simulink model "MORUS_NELINEARNI_GA_NONTILTING"  (R2019a)
settings: Solver=FixedStepAuto  StartTime=0.0  StopTime=sim_time  RelTol=1e-3  EnableMultiTasking=on
values from neighbouring files (symbols this model uses):
  A_dis_calc = expm(kSamplingTime*A_continous_time)    [MPC_designer_X.m]    (also in NonTilting.m; RUN_simulation.m; Simulacija_MPC_YAW_NELINEARNI.m; Simulacija_MPC_Z.m)
  B_dis_calc = integral_exp_A * B_continous_time    [MPC_designer_X.m]    (also in NonTilting.m; RUN_simulation.m; Simulacija_MPC_YAW_NELINEARNI.m; Simulacija_MPC_Z.m)
  b_f = 4.56e-4    (= 0.000456)    [LinearizacijaMatrica.m]    (also in Linearizirane_matrice.mat; MPC_designer_X.m; NonTilting.m; RUN_simulation.m)
  b_m = 0.01    [LinearizacijaMatrica.m]    (also in Linearizirane_matrice.mat; MPC_designer_X.m; NonTilting.m; RUN_simulation.m)
  BETA = 0.0    (= 0)    [LinearizacijaMatrica.m]    (also in Linearizirane_matrice.mat; MPC_designer_X.m; NonTilting.m = 0.200712863979; RUN_simulation.m)
  g = 9.80665    [LinearizacijaMatrica.m]    (also in Linearizirane_matrice.mat; MPC_designer_X.m = 9.81; NonTilting.m = 9.81; RUN_simulation.m = 9.81)
  hover = 427.6233    [MPC_designer_X.m]    (also in NonTilting.m; RUN_simulation.m; Simulacija_MPC_YAW_NELINEARNI.m; Simulacija_MPC_Z.m)
  I_b_xx = 5.5268    [MPC_designer_X.m]    (also in NonTilting.m; RUN_simulation.m; Simulacija_MPC_YAW_NELINEARNI.m; Simulacija_MPC_Z.m)
  I_b_yy = 5.5268    [MPC_designer_X.m]    (also in NonTilting.m; RUN_simulation.m; Simulacija_MPC_YAW_NELINEARNI.m; Simulacija_MPC_Z.m)
  I_b_zz = 6.8854    [MPC_designer_X.m]    (also in NonTilting.m; RUN_simulation.m; Simulacija_MPC_YAW_NELINEARNI.m; Simulacija_MPC_Z.m)
  kSamplingTime = 0.810    (= 0.81)    [MPCDesigner_YAW.m]    (also in MPC_designer_X.m = 0.1; MPC_designer_Z.m; NonTilting.m = 0.015; RUN_simulation.m = 0.015)
  L = 0.84    [LinearizacijaMatrica.m]    (also in Linearizirane_matrice.mat; MPC_designer_X.m; NonTilting.m; RUN_simulation.m)
  m = 1.0    (= 1)    [LinearizacijaMatrica.m]    (also in Linearizirane_matrice.mat; MPC_designer_X.m; NonTilting.m; RUN_simulation.m)
  M = 34.8    [LinearizacijaMatrica.m]    (also in Linearizirane_matrice.mat; MPC_designer_X.m = 34; NonTilting.m = 34; RUN_simulation.m = 34)
  m_b = 30.8    [LinearizacijaMatrica.m]    (also in Linearizirane_matrice.mat; MPC_designer_X.m; NonTilting.m; RUN_simulation.m)
  odabir = 1    [MPC_designer_X.m]    (also in NonTilting.m; RUN_simulation.m; Simulacija_MPC_YAW_NELINEARNI.m; Simulacija_MPC_Z.m)
  Q = inv(diag([0.5800 4*kSamplingTime 0.5800 4*kSamplingTime 300 300 0.2 (0.2/3) 100 4])) * diag([0, 0, 0, 0, 0, 0, 1e5,0, 1e7, 0]) *inv(diag([0.5800 4*kSamplingTime 0.5800 4*kSamplingTime 300 300 0.2 (0.2/3.0) 100 4]))    [NonTilting.m]    (also in RUN_simulation.m = diag([ 0.135340000000000,0.002706800000000,  0.1353400, 0.00; Simulacija_MPC_YAW_NELINEARNI.m = diag([pop(5),pop(6),pop(5),pop(6), pop(7),pop(7),pop(8),pop(; Simulacija_MPC_Z.m = diag([pop(5),pop(6),pop(5),pop(6), pop(7),pop(7),pop(8),pop(; Simulacija_Roll.m = diag([pop(5),pop(6),pop(5),pop(6), pop(7),pop(7),pop(8),pop()
  R = inv(diag([0.5800 0.5800 300 300]))*diag([0, 0, 0, 0])*inv(diag([0.5800 0.5800 300 300]))    [NonTilting.m]    (also in RUN_simulation.m = diag([0.67670, 0.67670, 0.13534000, 0.13534000]); Simulacija_MPC_YAW_NELINEARNI.m = diag([pop(1),pop(1),pop(2),pop(2)]); Simulacija_MPC_Z.m = diag([pop(1),pop(1),pop(2),pop(2)]); Simulacija_Roll.m = diag([pop(1),pop(1),pop(2),pop(2)]))
  R_delta = inv(diag([0.5800 0.5800 300 300]))* diag([0,0,0,0])*inv(diag([0.5800 0.5800 300 300]))    [NonTilting.m]    (also in RUN_simulation.m = diag([0.738879858135067, 0.738879858135067, 0.00738879858135; Simulacija_MPC_YAW_NELINEARNI.m = diag([pop(3),pop(3),pop(4),pop(4)]); Simulacija_MPC_Z.m = diag([pop(3),pop(3),pop(4),pop(4)]); Simulacija_Roll.m = diag([pop(3),pop(3),pop(4),pop(4)]))
  T_r = 0.2    [LinearizacijaMatrica.m]    (also in Linearizirane_matrice.mat; MPC_designer_X.m; NonTilting.m; RUN_simulation.m)
  w_mm = 19.7845    [LinearizacijaMatrica.m]    (also in Linearizirane_matrice.mat; MPC_designer_X.m = 17; NonTilting.m = 17; RUN_simulation.m = 17)
  z_m = 0.05    [LinearizacijaMatrica.m]    (also in Linearizirane_matrice.mat; MPC_designer_X.m; NonTilting.m; RUN_simulation.m)
  z_r = 0.2    [LinearizacijaMatrica.m]    (also in Linearizirane_matrice.mat; MPC_designer_X.m; NonTilting.m; RUN_simulation.m)
  zeta_mm = 0.6544    [LinearizacijaMatrica.m]    (also in Linearizirane_matrice.mat; MPC_designer_X.m = 0.85; NonTilting.m = 0.85; RUN_simulation.m = 0.85)
libraries: simulink x8
(part 3 of 4)

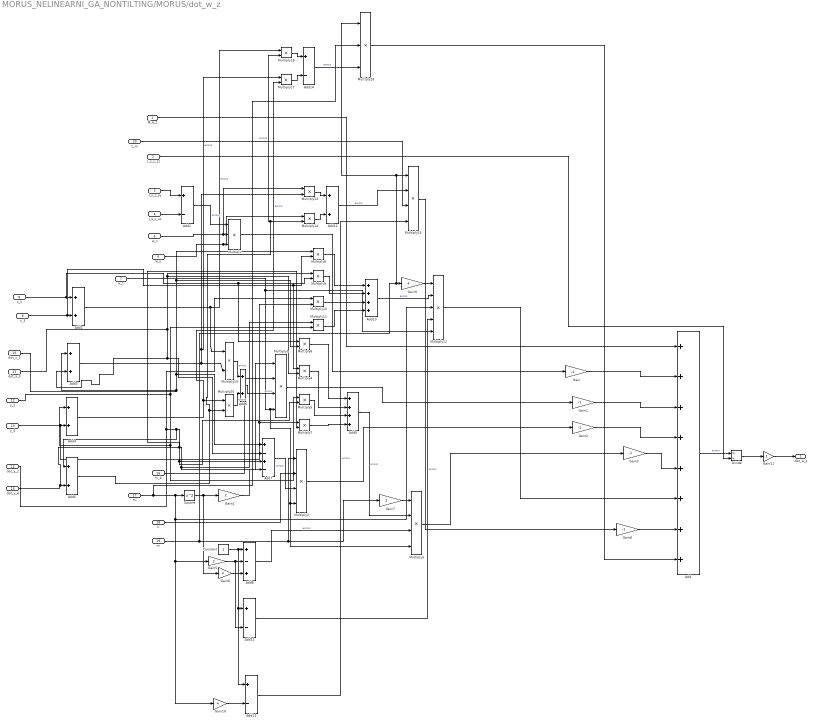
== system MORUS_NELINEARNI_GA_NONTILTING/MORUS/dot_w_z ==
  M_e_z : Inport
  I_s_c_zz : Inport  Port=2
  I_s_c_yy : Inport  Port=3
  I_s_c_xx : Inport  Port=4
  w_x : Inport  Port=5
  w_y : Inport  Port=6
  w_z : Inport  Port=7
  x_1 : Inport  Port=8
  x_3 : Inport  Port=9
  dot_x_1 : Inport  Port=10
  dot_x_3 : Inport  Port=11
  y_2 : Inport  Port=12
  y_4 : Inport  Port=13
  dot_y_2 : Inport  Port=14
  dot_y_4 : Inport  Port=15
  m_b : Inport  Port=16
  mi : Inport  Port=17
  L : Inport  Port=18
  m : Inport  Port=19
  z_m : Inport  Port=20
  Add : Sum  Inputs=++++++++  AccumDataTypeStr=double  OutDataTypeStr=double
  Add{1,11,13..14} (4 alike) : Sum  Inputs=+-  AccumDataTypeStr=double  OutDataTypeStr=double
  Add10 : Sum  Inputs=++++  AccumDataTypeStr=double  OutDataTypeStr=double
  Add{2..6,12} (6 alike) : Sum  AccumDataTypeStr=double  OutDataTypeStr=double
  Add7 : Sum  Inputs=+-+-  AccumDataTypeStr=double  OutDataTypeStr=double
  Add8 : Sum  Inputs=+-+  AccumDataTypeStr=double  OutDataTypeStr=double
  Add9 : Sum  Inputs=++++  AccumDataTypeStr=double  OutDataTypeStr=double
  Constant : Constant  OutDataTypeStr=double  SampleTime=-1
  Divide : Product  Inputs=*/  OutDataTypeStr=double
  Gain{,1..3,8} (5 alike) : Gain  Gain=-1
  Gain10 : Gain  Gain=4
  Gain11 : Gain
  Gain4 : Gain  Gain=2
  Gain5 : Gain  Gain=2
  Gain6 : Gain  Gain=4
  Gain7 : Gain  Gain=2
  Gain9 : Gain  Gain=4
  Multiply : Product  Inputs=3
  Multiply{1..3,15} (4 alike) : Product  Inputs=4
  Multiply{4..11,13..14,16..17,19..20} (14 alike) : Product
  Multiply12 : Product  Inputs=5
  Multiply18 : Product  Inputs=3
  Square : Math  Operator=square  SaturateOnIntegerOverflow=on
  dot_w_z : Outport  OutDataTypeStr=double
  wires:
  Add/1 -> Divide/1  "errors"
  I_s_c_zz/1 -> Divide/2
  Divide/1 -> Gain11/1
  M_e_z/1 -> Add/1
  I_s_c_xx/1 -> Add1/2
  I_s_c_yy/1 -> Add1/1
  Add1/1 -> Multiply/1  "errors"
  w_x/1 -> Multiply13/1, Multiply/2
  w_y/1 -> Multiply14/1, Multiply/3
  Gain/1 -> Add/2
  Gain2/1 -> Add/4
  Gain1/1 -> Add/3
  Gain3/1 -> Add/5
  Multiply/1 -> Gain/1
  x_1/1 -> Multiply6/1, Multiply9/2, Add2/1
  x_3/1 -> Multiply4/1, Multiply8/2, Add2/2
  dot_x_1/1 -> Multiply6/2, Multiply8/1, Add7/1, Add3/1
  dot_x_3/1 -> Add7/2, Add3/2, Multiply4/2, Multiply9/1
  y_4/1 -> Multiply7/1, Multiply10/2, Add4/2
  y_2/1 -> Multiply5/1, Add4/1, Multiply11/2
  dot_y_2/1 -> Add7/3, Multiply5/2, Add5/1, Multiply10/1
  dot_y_4/1 -> Add7/4, Multiply11/1, Multiply7/2, Add5/2
  Add2/1 -> Multiply19/1, Multiply16/1  "errors"
  Add3/1 -> Multiply19/2, Multiply17/1, Multiply13/2  "errors"
  Add4/1 -> Multiply20/1, Multiply17/2  "errors"
  Add5/1 -> Multiply14/2, Multiply16/2, Multiply20/2  "errors"
  w_z/1 -> Multiply12/5, Multiply3/4, Multiply2/4, Multiply1/4
  mi/1 -> Multiply18/2, Gain10/1, Gain5/1, Multiply12/3, Square/1
  m_b/1 -> Multiply1/2
  Square/1 -> Gain6/1, Gain4/1
  Gain4/1 -> Multiply1/1
  Multiply1/1 -> Gain1/1
  Add7/1 -> Multiply2/3  "errors"
  m/1 -> Multiply18/1, Multiply15/1, Gain9/1, Gain7/1, Multiply2/1
  L/1 -> Multiply2/2
  Multiply2/1 -> Gain2/1
  Gain5/1 -> Add8/2, Add11/2
  Gain6/1 -> Add8/3
  Constant/1 -> Add13/1, Add11/1, Add8/1
  Add8/1 -> Multiply3/3  "errors"
  Gain7/1 -> Multiply3/1
  Multiply3/1 -> Gain3/1
  Multiply6/1 -> Add9/1
  Multiply4/1 -> Add9/2
  Multiply5/1 -> Add9/3
  Multiply7/1 -> Add9/4
  Add9/1 -> Multiply3/2  "errors"
  Gain8/1 -> Add/7
  Multiply8/1 -> Add10/1
  Multiply9/1 -> Add10/2
  Multiply10/1 -> Add10/3
  Multiply11/1 -> Add10/4
  Gain9/1 -> Multiply12/1
  Add10/1 -> Multiply12/2  "errors"
  Add11/1 -> Multiply12/4  "errors"
  Multiply12/1 -> Add/6
  Multiply13/1 -> Add12/1
  Multiply14/1 -> Add12/2
  Add12/1 -> Multiply15/2  "errors"
  z_m/1 -> Multiply15/3
  Gain10/1 -> Add13/2
  Add13/1 -> Multiply15/4  "errors"
  Multiply15/1 -> Gain8/1
  Multiply17/1 -> Add14/2
  Multiply16/1 -> Add14/1
  Add14/1 -> Multiply18/3  "errors"
  Multiply18/1 -> Add/8
  Multiply19/1 -> Add6/1  "errors"
  Multiply20/1 -> Add6/2  "errors"
  Add6/1 -> Multiply1/3  "errors"
  Gain11/1 -> dot_w_z/1

== system MORUS_NELINEARNI_GA_NONTILTING/MORUS/I_1_c/I_11 ==
  y2 : Inport
  y4 : Inport  Port=2
  m : Inport  Port=3
  mi : Inport  Port=4
  z_m : Inport  Port=5
  Constant : Constant  OutDataTypeStr=double  SampleTime=-1
  Gain : Gain  Gain=4
  Multiply : Product
  Multiply1 : Product  OutDataTypeStr=double
  Multiply2 : Product
  Square : Math  Operator=square  SaturateOnIntegerOverflow=on
  Square1 : Math  Operator=square  SaturateOnIntegerOverflow=on
  Sum : Sum
  Sum1 : Sum
  Sum2 : Sum  Inputs=+-
  I_11 : Outport
  wires:
  Multiply1/1 -> I_11/1
  y2/1 -> Sum/1
  y4/1 -> Sum/2
  Sum/1 -> Multiply/1
  mi/1 -> Gain/1, Multiply/2
  Multiply/1 -> Square/1
  Square/1 -> Sum1/1
  m/1 -> Multiply1/1
  Sum1/1 -> Multiply1/2
  Gain/1 -> Sum2/2
  Sum2/1 -> Multiply2/2
  Multiply2/1 -> Square1/1
  Square1/1 -> Sum1/2
  Constant/1 -> Sum2/1
  z_m/1 -> Multiply2/1

== system MORUS_NELINEARNI_GA_NONTILTING/MORUS/I_1_c/I_12 // I_21 ==
  m : Inport
  mi : Inport  Port=2
  x_1 : Inport  Port=3
  x_3 : Inport  Port=4
  y_2 : Inport  Port=5
  y_4 : Inport  Port=6
  L : Inport  Port=7
  Gain : Gain  Gain=0.5
  Multiply : Product  Inputs=4
  Multiply1 : Product
  Sum : Sum
  Sum1 : Sum
  Sum2 : Sum  Inputs=+-+
  I_12 : Outport
  wires:
  y_2/1 -> Sum1/1
  y_4/1 -> Sum1/2
  x_3/1 -> Sum/2
  x_1/1 -> Sum2/1, Sum/1
  Multiply/1 -> I_12/1
  m/1 -> Multiply/1
  mi/1 -> Multiply1/1, Multiply/2
  Sum1/1 -> Multiply/4
  Sum/1 -> Multiply1/2
  Multiply1/1 -> Sum2/2
  Sum2/1 -> Multiply/3
  L/1 -> Gain/1
  Gain/1 -> Sum2/3

== system MORUS_NELINEARNI_GA_NONTILTING/MORUS/I_1_c/I_13 // I_31 ==
  m : Inport
  mi : Inport  Port=2
  x_1 : Inport  Port=3
  x_3 : Inport  Port=4
  L : Inport  Port=5
  z_m : Inport  Port=6
  Constant : Constant  OutDataTypeStr=double  SampleTime=-1
  Gain : Gain  Gain=0.5
  Gain1 : Gain  Gain=-1
  Gain2 : Gain  Gain=4
  Multiply : Product  Inputs=3
  Multiply1 : Product
  Multiply2 : Product
  Sum : Sum
  Sum2 : Sum  Inputs=+-+
  Sum3 : Sum  Inputs=+-
  I_13 : Outport
  wires:
  m/1 -> Gain1/1
  mi/1 -> Multiply1/1, Gain2/1
  Sum/1 -> Multiply1/2
  L/1 -> Gain/1
  Multiply/1 -> I_13/1
  Gain/1 -> Sum2/3
  Sum2/1 -> Multiply/2
  x_1/1 -> Sum2/1, Sum/1
  x_3/1 -> Sum/2
  Multiply1/1 -> Sum2/2
  Gain1/1 -> Multiply/1
  Gain2/1 -> Sum3/2
  Sum3/1 -> Multiply2/2
  Constant/1 -> Sum3/1
  z_m/1 -> Multiply2/1
  Multiply2/1 -> Multiply/3

== system MORUS_NELINEARNI_GA_NONTILTING/MORUS/I_1_c/I_22 ==
  x1 : Inport
  x3 : Inport  Port=2
  m : Inport  Port=3
  mi : Inport  Port=4
  z_m : Inport  Port=5
  L : Inport  Port=6
  Constant : Constant  OutDataTypeStr=double  SampleTime=-1
  Gain : Gain  Gain=4
  Gain1 : Gain  Gain=0.5
  Multiply : Product
  Multiply1 : Product
  Multiply2 : Product
  Square : Math  Operator=square  SaturateOnIntegerOverflow=on
  Square1 : Math  Operator=square  SaturateOnIntegerOverflow=on
  Sum : Sum
  Sum1 : Sum
  Sum2 : Sum  Inputs=+-
  Sum3 : Sum  Inputs=-++
  I_22 : Outport
  wires:
  Gain/1 -> Sum2/2
  mi/1 -> Multiply/2, Gain/1
  Sum/1 -> Multiply/1
  Sum1/1 -> Multiply1/2
  x3/1 -> Sum/2
  Multiply2/1 -> Square1/1
  Constant/1 -> Sum2/1
  Sum2/1 -> Multiply2/2
  Square/1 -> Sum1/1
  Sum3/1 -> Square/1
  z_m/1 -> Multiply2/1
  Multiply1/1 -> I_22/1
  m/1 -> Multiply1/1
  Square1/1 -> Sum1/2
  x1/1 -> Sum3/2, Sum/1
  Multiply/1 -> Sum3/1
  L/1 -> Gain1/1
  Gain1/1 -> Sum3/3

== system MORUS_NELINEARNI_GA_NONTILTING/MORUS/I_1_c/I_23 // I_32 ==
  m : Inport
  mi : Inport  Port=2
  y_2 : Inport  Port=3
  y_4 : Inport  Port=4
  z_m : Inport  Port=5
  Constant : Constant  OutDataTypeStr=double  SampleTime=-1
  Gain : Gain  Gain=4
  Multiply : Product  Inputs=5
  Sum : Sum
  Sum1 : Sum  Inputs=+-
  I_23 : Outport
  wires:
  z_m/1 -> Multiply/4
  y_4/1 -> Sum/2
  y_2/1 -> Sum/1
  Multiply/1 -> I_23/1
  m/1 -> Multiply/1
  mi/1 -> Gain/1, Multiply/2
  Sum/1 -> Multiply/3
  Sum1/1 -> Multiply/5
  Gain/1 -> Sum1/2
  Constant/1 -> Sum1/1

== system MORUS_NELINEARNI_GA_NONTILTING/MORUS/I_1_c/I_33 ==
  x1 : Inport
  x3 : Inport  Port=2
  m : Inport  Port=3
  mi : Inport  Port=4
  L : Inport  Port=5
  y2 : Inport  Port=6
  y4 : Inport  Port=7
  Gain1 : Gain  Gain=0.5
  Multiply : Product
  Multiply1 : Product
  Multiply2 : Product
  Square : Math  Operator=square  SaturateOnIntegerOverflow=on
  Square1 : Math  Operator=square  SaturateOnIntegerOverflow=on
  Sum : Sum
  Sum1 : Sum
  Sum2 : Sum
  Sum3 : Sum  Inputs=-++
  I_33 : Outport
  wires:
  Multiply1/1 -> I_33/1
  m/1 -> Multiply1/1
  Multiply2/1 -> Square1/1
  x3/1 -> Sum/2
  mi/1 -> Multiply2/1, Multiply/2
  Multiply/1 -> Sum3/1
  Sum1/1 -> Multiply1/2
  x1/1 -> Sum3/2, Sum/1
  Sum/1 -> Multiply/1
  Square/1 -> Sum1/1
  Gain1/1 -> Sum3/3
  Square1/1 -> Sum1/2
  L/1 -> Gain1/1
  Sum3/1 -> Square/1
  y2/1 -> Sum2/1
  y4/1 -> Sum2/2
  Sum2/1 -> Multiply2/2

== system MORUS_NELINEARNI_GA_NONTILTING/MORUS/I_2_c/I_11 ==
  y2 : Inport
  y4 : Inport  Port=2
  m : Inport  Port=3
  mi : Inport  Port=4
  z_m : Inport  Port=5
  L : Inport  Port=6
  Constant : Constant  OutDataTypeStr=double  SampleTime=-1
  Gain : Gain  Gain=4
  Gain1 : Gain  Gain=0.5
  Multiply : Product
  Multiply1 : Product
  Multiply2 : Product
  Square : Math  Operator=square  SaturateOnIntegerOverflow=on
  Square1 : Math  Operator=square  SaturateOnIntegerOverflow=on
  Sum : Sum
  Sum1 : Sum
  Sum2 : Sum  Inputs=+-
  Sum3 : Sum  Inputs=-++
  I_11 : Outport
  wires:
  Gain/1 -> Sum2/2
  mi/1 -> Multiply/2, Gain/1
  Sum/1 -> Multiply/1
  Sum1/1 -> Multiply1/2
  y4/1 -> Sum/2
  Multiply2/1 -> Square1/1
  Constant/1 -> Sum2/1
  Sum2/1 -> Multiply2/2
  Square/1 -> Sum1/1
  Sum3/1 -> Square/1
  z_m/1 -> Multiply2/1
  Multiply1/1 -> I_11/1
  m/1 -> Multiply1/1
  Square1/1 -> Sum1/2
  y2/1 -> Sum3/2, Sum/1
  Multiply/1 -> Sum3/1
  L/1 -> Gain1/1
  Gain1/1 -> Sum3/3

== system MORUS_NELINEARNI_GA_NONTILTING/MORUS/I_2_c/I_12 // I_21 ==
  m : Inport
  mi : Inport  Port=2
  y2 : Inport  Port=3
  y4 : Inport  Port=4
  x1 : Inport  Port=5
  x3 : Inport  Port=6
  L : Inport  Port=7
  Gain : Gain  Gain=0.5
  Multiply : Product  Inputs=4
  Multiply1 : Product
  Sum : Sum
  Sum1 : Sum
  Sum2 : Sum  Inputs=+-+
  I_12 : Outport
  wires:
  x1/1 -> Sum1/1
  x3/1 -> Sum1/2
  y4/1 -> Sum/2
  y2/1 -> Sum2/1, Sum/1
  Multiply/1 -> I_12/1
  m/1 -> Multiply/1
  mi/1 -> Multiply1/1, Multiply/2
  Sum1/1 -> Multiply/4
  Sum/1 -> Multiply1/2
  Multiply1/1 -> Sum2/2
  Sum2/1 -> Multiply/3
  L/1 -> Gain/1
  Gain/1 -> Sum2/3

== system MORUS_NELINEARNI_GA_NONTILTING/MORUS/I_2_c/I_13 // I_31_ ==
  m : Inport
  mi : Inport  Port=2
  x1 : Inport  Port=3
  x3 : Inport  Port=4
  z_m : Inport  Port=5
  Constant : Constant  OutDataTypeStr=double  SampleTime=-1
  Gain : Gain  Gain=4
  Multiply : Product  Inputs=5
  Sum : Sum
  Sum1 : Sum  Inputs=+-
  I_13 : Outport
  wires:
  z_m/1 -> Multiply/4
  x3/1 -> Sum/2
  x1/1 -> Sum/1
  Multiply/1 -> I_13/1
  m/1 -> Multiply/1
  mi/1 -> Gain/1, Multiply/2
  Sum/1 -> Multiply/3
  Sum1/1 -> Multiply/5
  Gain/1 -> Sum1/2
  Constant/1 -> Sum1/1

== system MORUS_NELINEARNI_GA_NONTILTING/MORUS/I_2_c/I_22 ==
  x1 : Inport
  x3 : Inport  Port=2
  m : Inport  Port=3
  mi : Inport  Port=4
  z_m : Inport  Port=5
  Constant : Constant  OutDataTypeStr=double  SampleTime=-1
  Gain : Gain  Gain=4
  Multiply : Product
  Multiply1 : Product  OutDataTypeStr=double
  Multiply2 : Product
  Square : Math  Operator=square  SaturateOnIntegerOverflow=on
  Square1 : Math  Operator=square  SaturateOnIntegerOverflow=on
  Sum : Sum
  Sum1 : Sum
  Sum2 : Sum  Inputs=+-
  I_22 : Outport
  wires:
  Multiply1/1 -> I_22/1
  x1/1 -> Sum/1
  x3/1 -> Sum/2
  Sum/1 -> Multiply/1
  mi/1 -> Gain/1, Multiply/2
  Multiply/1 -> Square/1
  Square/1 -> Sum1/1
  m/1 -> Multiply1/1
  Sum1/1 -> Multiply1/2
  Gain/1 -> Sum2/2
  Sum2/1 -> Multiply2/2
  Multiply2/1 -> Square1/1
  Square1/1 -> Sum1/2
  Constant/1 -> Sum2/1
  z_m/1 -> Multiply2/1

== system MORUS_NELINEARNI_GA_NONTILTING/MORUS/I_2_c/I_23 // I_32 ==
  m : Inport
  mi : Inport  Port=2
  y2 : Inport  Port=3
  y4 : Inport  Port=4
  L : Inport  Port=5
  z_m : Inport  Port=6
  Constant : Constant  OutDataTypeStr=double  SampleTime=-1
  Gain : Gain  Gain=0.5
  Gain1 : Gain  Gain=-1
  Gain2 : Gain  Gain=4
  Multiply : Product  Inputs=4
  Multiply1 : Product
  Multiply2 : Product
  Sum : Sum
  Sum2 : Sum  Inputs=+-+
  Sum3 : Sum  Inputs=+-
  I_23 : Outport
  wires:
  m/1 -> Gain1/1
  mi/1 -> Multiply1/1, Gain2/1, Multiply/4
  Sum/1 -> Multiply1/2
  L/1 -> Gain/1
  Multiply/1 -> I_23/1
  Gain/1 -> Sum2/3
  Sum2/1 -> Multiply/2
  y2/1 -> Sum2/1, Sum/1
  y4/1 -> Sum/2
  Multiply1/1 -> Sum2/2
  Gain1/1 -> Multiply/1
  Gain2/1 -> Sum3/2
  Sum3/1 -> Multiply2/2
  Constant/1 -> Sum3/1
  z_m/1 -> Multiply2/1
  Multiply2/1 -> Multiply/3

== system MORUS_NELINEARNI_GA_NONTILTING/MORUS/I_2_c/I_33 ==
  y2 : Inport
  y4 : Inport  Port=2
  m : Inport  Port=3
  mi : Inport  Port=4
  L : Inport  Port=5
  x1 : Inport  Port=6
  x3 : Inport  Port=7
  Gain1 : Gain  Gain=0.5
  Multiply : Product
  Multiply1 : Product
  Multiply2 : Product
  Square : Math  Operator=square  SaturateOnIntegerOverflow=on
  Square1 : Math  Operator=square  SaturateOnIntegerOverflow=on
  Sum : Sum
  Sum1 : Sum
  Sum2 : Sum
  Sum3 : Sum  Inputs=-++
  I_33 : Outport
  wires:
  Multiply1/1 -> I_33/1
  m/1 -> Multiply1/1
  Multiply2/1 -> Square1/1
  y4/1 -> Sum/2
  mi/1 -> Multiply2/1, Multiply/2
  Multiply/1 -> Sum3/1
  Sum1/1 -> Multiply1/2
  y2/1 -> Sum3/2, Sum/1
  Sum/1 -> Multiply/1
  Square/1 -> Sum1/1
  Gain1/1 -> Sum3/3
  Square1/1 -> Sum1/2
  L/1 -> Gain1/1
  Sum3/1 -> Square/1
  x1/1 -> Sum2/1
  x3/1 -> Sum2/2
  Sum2/1 -> Multiply2/2

== system MORUS_NELINEARNI_GA_NONTILTING/MORUS/I_3_c/I_11 ==
  y2 : Inport
  y4 : Inport  Port=2
  m : Inport  Port=3
  mi : Inport  Port=4
  z_m : Inport  Port=5
  Constant : Constant  OutDataTypeStr=double  SampleTime=-1
  Gain : Gain  Gain=4
  Multiply : Product
  Multiply1 : Product
  Multiply2 : Product
  Square : Math  Operator=square  SaturateOnIntegerOverflow=on
  Square1 : Math  Operator=square  SaturateOnIntegerOverflow=on
  Sum : Sum
  Sum1 : Sum
  Sum2 : Sum  Inputs=+-
  I_11 : Outport
  wires:
  Multiply1/1 -> I_11/1
  y2/1 -> Sum/1
  y4/1 -> Sum/2
  Sum/1 -> Multiply/1
  mi/1 -> Gain/1, Multiply/2
  Multiply/1 -> Square/1
  Square/1 -> Sum1/1
  m/1 -> Multiply1/1
  Sum1/1 -> Multiply1/2
  Gain/1 -> Sum2/2
  Sum2/1 -> Multiply2/2
  Multiply2/1 -> Square1/1
  Square1/1 -> Sum1/2
  Constant/1 -> Sum2/1
  z_m/1 -> Multiply2/1

== system MORUS_NELINEARNI_GA_NONTILTING/MORUS/I_3_c/I_12 // I_21 ==
  m : Inport
  mi : Inport  Port=2
  x_1 : Inport  Port=3
  x_3 : Inport  Port=4
  y_2 : Inport  Port=5
  y_4 : Inport  Port=6
  L : Inport  Port=7
  Gain : Gain  Gain=-0.5
  Multiply : Product  Inputs=4
  Multiply1 : Product
  Sum : Sum
  Sum1 : Sum
  Sum2 : Sum  Inputs=+-+
  I_12 : Outport
  wires:
  y_2/1 -> Sum1/1
  y_4/1 -> Sum1/2
  x_3/1 -> Sum2/1, Sum/2
  x_1/1 -> Sum/1
  Multiply/1 -> I_12/1
  m/1 -> Multiply/1
  mi/1 -> Multiply1/1, Multiply/2
  Sum1/1 -> Multiply/4
  Sum/1 -> Multiply1/2
  Multiply1/1 -> Sum2/2
  Sum2/1 -> Multiply/3
  L/1 -> Gain/1
  Gain/1 -> Sum2/3

== system MORUS_NELINEARNI_GA_NONTILTING/MORUS/I_3_c/I_13 // I_31 ==
  m : Inport
  mi : Inport  Port=2
  x_1 : Inport  Port=3
  x_3 : Inport  Port=4
  L : Inport  Port=5
  z_m : Inport  Port=6
  Constant : Constant  OutDataTypeStr=double  SampleTime=-1
  Gain : Gain  Gain=-0.5
  Gain1 : Gain  Gain=-1
  Gain2 : Gain  Gain=4
  Multiply : Product  Inputs=3
  Multiply1 : Product
  Multiply2 : Product
  Sum : Sum
  Sum2 : Sum  Inputs=+-+
  Sum3 : Sum  Inputs=+-
  I_13 : Outport
  wires:
  m/1 -> Gain1/1
  mi/1 -> Multiply1/1, Gain2/1
  Sum/1 -> Multiply1/2
  L/1 -> Gain/1
  Multiply/1 -> I_13/1
  Gain/1 -> Sum2/3
  Sum2/1 -> Multiply/2
  x_1/1 -> Sum/1
  x_3/1 -> Sum2/1, Sum/2
  Multiply1/1 -> Sum2/2
  Gain1/1 -> Multiply/1
  Gain2/1 -> Sum3/2
  Sum3/1 -> Multiply2/2
  Constant/1 -> Sum3/1
  z_m/1 -> Multiply2/1
  Multiply2/1 -> Multiply/3

== system MORUS_NELINEARNI_GA_NONTILTING/MORUS/I_3_c/I_22 ==
  x1 : Inport
  x3 : Inport  Port=2
  m : Inport  Port=3
  mi : Inport  Port=4
  z_m : Inport  Port=5
  L : Inport  Port=6
  Constant : Constant  OutDataTypeStr=double  SampleTime=-1
  Gain : Gain  Gain=4
  Gain1 : Gain  Gain=-0.5
  Multiply : Product
  Multiply1 : Product
  Multiply2 : Product
  Square : Math  Operator=square  SaturateOnIntegerOverflow=on
  Square1 : Math  Operator=square  SaturateOnIntegerOverflow=on
  Sum : Sum
  Sum1 : Sum
  Sum2 : Sum  Inputs=+-
  Sum3 : Sum  Inputs=-++
  I_22 : Outport
  wires:
  Gain/1 -> Sum2/2
  mi/1 -> Multiply/2, Gain/1
  Sum/1 -> Multiply/1
  Sum1/1 -> Multiply1/2
  x3/1 -> Sum/2, Sum3/2
  Multiply2/1 -> Square1/1
  Constant/1 -> Sum2/1
  Sum2/1 -> Multiply2/2
  Square/1 -> Sum1/1
  Sum3/1 -> Square/1
  z_m/1 -> Multiply2/1
  Multiply1/1 -> I_22/1
  m/1 -> Multiply1/1
  Square1/1 -> Sum1/2
  x1/1 -> Sum/1
  Multiply/1 -> Sum3/1
  L/1 -> Gain1/1
  Gain1/1 -> Sum3/3

== system MORUS_NELINEARNI_GA_NONTILTING/MORUS/I_3_c/I_23 // I_32 ==
  m : Inport
  mi : Inport  Port=2
  y_2 : Inport  Port=3
  y_4 : Inport  Port=4
  z_m : Inport  Port=5
  Constant : Constant  OutDataTypeStr=double  SampleTime=-1
  Gain : Gain  Gain=4
  Multiply : Product  Inputs=5
  Sum : Sum
  Sum1 : Sum  Inputs=+-
  I_23 : Outport
  wires:
  z_m/1 -> Multiply/4
  y_4/1 -> Sum/2
  y_2/1 -> Sum/1
  Multiply/1 -> I_23/1
  m/1 -> Multiply/1
  mi/1 -> Gain/1, Multiply/2
  Sum/1 -> Multiply/3
  Sum1/1 -> Multiply/5
  Gain/1 -> Sum1/2
  Constant/1 -> Sum1/1

== system MORUS_NELINEARNI_GA_NONTILTING/MORUS/I_3_c/I_33 ==
  x1 : Inport
  x3 : Inport  Port=2
  m : Inport  Port=3
  mi : Inport  Port=4
  L : Inport  Port=5
  y2 : Inport  Port=6
  y4 : Inport  Port=7
  Gain1 : Gain  Gain=-0.5
  Multiply : Product
  Multiply1 : Product
  Multiply2 : Product
  Square : Math  Operator=square  SaturateOnIntegerOverflow=on
  Square1 : Math  Operator=square  SaturateOnIntegerOverflow=on
  Sum : Sum
  Sum1 : Sum
  Sum2 : Sum
  Sum3 : Sum  Inputs=-++
  I_33 : Outport
  wires:
  Multiply1/1 -> I_33/1
  m/1 -> Multiply1/1
  Multiply2/1 -> Square1/1
  x3/1 -> Sum3/2, Sum/2
  mi/1 -> Multiply2/1, Multiply/2
  Multiply/1 -> Sum3/1
  Sum1/1 -> Multiply1/2
  x1/1 -> Sum/1
  Sum/1 -> Multiply/1
  Square/1 -> Sum1/1
  Gain1/1 -> Sum3/3
  Square1/1 -> Sum1/2
  L/1 -> Gain1/1
  Sum3/1 -> Square/1
  y2/1 -> Sum2/1
  y4/1 -> Sum2/2
  Sum2/1 -> Multiply2/2

== system MORUS_NELINEARNI_GA_NONTILTING/MORUS/I_4_c/I_11 ==
  y2 : Inport
  y4 : Inport  Port=2
  m : Inport  Port=3
  mi : Inport  Port=4
  z_m : Inport  Port=5
  L : Inport  Port=6
  Constant : Constant  OutDataTypeStr=double  SampleTime=-1
  Gain : Gain  Gain=4
  Gain1 : Gain  Gain=-0.5
  Multiply : Product
  Multiply1 : Product
  Multiply2 : Product
  Square : Math  Operator=square  SaturateOnIntegerOverflow=on
  Square1 : Math  Operator=square  SaturateOnIntegerOverflow=on
  Sum : Sum
  Sum1 : Sum
  Sum2 : Sum  Inputs=+-
  Sum3 : Sum  Inputs=-++
  I_11 : Outport
  wires:
  Gain/1 -> Sum2/2
  mi/1 -> Multiply/2, Gain/1
  Sum/1 -> Multiply/1
  Sum1/1 -> Multiply1/2
  y4/1 -> Sum/2, Sum3/2
  Multiply2/1 -> Square1/1
  Constant/1 -> Sum2/1
  Sum2/1 -> Multiply2/2
  Square/1 -> Sum1/1
  Sum3/1 -> Square/1
  z_m/1 -> Multiply2/1
  Multiply1/1 -> I_11/1
  m/1 -> Multiply1/1
  Square1/1 -> Sum1/2
  y2/1 -> Sum/1
  Multiply/1 -> Sum3/1
  L/1 -> Gain1/1
  Gain1/1 -> Sum3/3

== system MORUS_NELINEARNI_GA_NONTILTING/MORUS/I_4_c/I_12 // I_21 ==
  m : Inport
  mi : Inport  Port=2
  y2 : Inport  Port=3
  y4 : Inport  Port=4
  x1 : Inport  Port=5
  x3 : Inport  Port=6
  L : Inport  Port=7
  Gain : Gain  Gain=-0.5
  Multiply : Product  Inputs=4
  Multiply1 : Product
  Sum : Sum
  Sum1 : Sum
  Sum2 : Sum  Inputs=+-+
  I_12 : Outport
  wires:
  x1/1 -> Sum1/1
  x3/1 -> Sum1/2
  y4/1 -> Sum2/1, Sum/2
  y2/1 -> Sum/1
  Multiply/1 -> I_12/1
  m/1 -> Multiply/1
  mi/1 -> Multiply1/1, Multiply/2
  Sum1/1 -> Multiply/4
  Sum/1 -> Multiply1/2
  Multiply1/1 -> Sum2/2
  Sum2/1 -> Multiply/3
  L/1 -> Gain/1
  Gain/1 -> Sum2/3

== system MORUS_NELINEARNI_GA_NONTILTING/MORUS/I_4_c/I_13 // I_31_ ==
  m : Inport
  mi : Inport  Port=2
  x1 : Inport  Port=3
  x3 : Inport  Port=4
  z_m : Inport  Port=5
  Constant : Constant  OutDataTypeStr=double  SampleTime=-1
  Gain : Gain  Gain=4
  Multiply : Product  Inputs=5
  Sum : Sum
  Sum1 : Sum  Inputs=+-
  I_13 : Outport
  wires:
  z_m/1 -> Multiply/4
  x3/1 -> Sum/2
  x1/1 -> Sum/1
  Multiply/1 -> I_13/1
  m/1 -> Multiply/1
  mi/1 -> Gain/1, Multiply/2
  Sum/1 -> Multiply/3
  Sum1/1 -> Multiply/5
  Gain/1 -> Sum1/2
  Constant/1 -> Sum1/1

== system MORUS_NELINEARNI_GA_NONTILTING/MORUS/I_4_c/I_22_ ==
  x1 : Inport
  x3 : Inport  Port=2
  m : Inport  Port=3
  mi : Inport  Port=4
  z_m : Inport  Port=5
  Constant : Constant  OutDataTypeStr=double  SampleTime=-1
  Gain : Gain  Gain=4
  Multiply : Product
  Multiply1 : Product
  Multiply2 : Product
  Square : Math  Operator=square  SaturateOnIntegerOverflow=on
  Square1 : Math  Operator=square  SaturateOnIntegerOverflow=on
  Sum : Sum
  Sum1 : Sum
  Sum2 : Sum  Inputs=+-
  I_22 : Outport
  wires:
  Multiply1/1 -> I_22/1
  x1/1 -> Sum/1
  x3/1 -> Sum/2
  Sum/1 -> Multiply/1
  mi/1 -> Gain/1, Multiply/2
  Multiply/1 -> Square/1
  Square/1 -> Sum1/1
  m/1 -> Multiply1/1
  Sum1/1 -> Multiply1/2
  Gain/1 -> Sum2/2
  Sum2/1 -> Multiply2/2
  Multiply2/1 -> Square1/1
  Square1/1 -> Sum1/2
  Constant/1 -> Sum2/1
  z_m/1 -> Multiply2/1

== system MORUS_NELINEARNI_GA_NONTILTING/MORUS/I_4_c/I_23 // I_32 ==
  m : Inport
  mi : Inport  Port=2
  y2 : Inport  Port=3
  y4 : Inport  Port=4
  L : Inport  Port=5
  z_m : Inport  Port=6
  Constant : Constant  OutDataTypeStr=double  SampleTime=-1
  Gain : Gain  Gain=-0.5
  Gain1 : Gain  Gain=-1
  Gain2 : Gain  Gain=4
  Multiply : Product  Inputs=4
  Multiply1 : Product
  Multiply2 : Product
  Sum : Sum
  Sum2 : Sum  Inputs=+-+
  Sum3 : Sum  Inputs=+-
  I_13 : Outport
  wires:
  m/1 -> Gain1/1
  mi/1 -> Multiply/4, Multiply1/1, Gain2/1
  Sum/1 -> Multiply1/2
  L/1 -> Gain/1
  Multiply/1 -> I_13/1
  Gain/1 -> Sum2/3
  Sum2/1 -> Multiply/2
  y2/1 -> Sum/1
  y4/1 -> Sum2/1, Sum/2
  Multiply1/1 -> Sum2/2
  Gain1/1 -> Multiply/1
  Gain2/1 -> Sum3/2
  Sum3/1 -> Multiply2/2
  Constant/1 -> Sum3/1
  z_m/1 -> Multiply2/1
  Multiply2/1 -> Multiply/3

== system MORUS_NELINEARNI_GA_NONTILTING/MORUS/I_4_c/I_33 ==
  y2 : Inport
  y4 : Inport  Port=2
  m : Inport  Port=3
  mi : Inport  Port=4
  L : Inport  Port=5
  x_1 : Inport  Port=6
  x_3 : Inport  Port=7
  Gain1 : Gain  Gain=-0.5
  Multiply : Product
  Multiply1 : Product
  Multiply2 : Product
  Square : Math  Operator=square  SaturateOnIntegerOverflow=on
  Square1 : Math  Operator=square  SaturateOnIntegerOverflow=on
  Sum : Sum
  Sum1 : Sum
  Sum2 : Sum
  Sum3 : Sum  Inputs=-++
  I_33 : Outport
  wires:
  Multiply1/1 -> I_33/1
  m/1 -> Multiply1/1
  Multiply2/1 -> Square1/1
  y4/1 -> Sum3/2, Sum/2
  mi/1 -> Multiply2/1, Multiply/2
  Multiply/1 -> Sum3/1
  Sum1/1 -> Multiply1/2
  y2/1 -> Sum/1
  Sum/1 -> Multiply/1
  Square/1 -> Sum1/1
  Gain1/1 -> Sum3/3
  Square1/1 -> Sum1/2
  L/1 -> Gain1/1
  Sum3/1 -> Square/1
  x_1/1 -> Sum2/1
  x_3/1 -> Sum2/2
  Sum2/1 -> Multiply2/2

== system MORUS_NELINEARNI_GA_NONTILTING/MORUS/I_b_c/I_11 ==
  I_b_xx : Inport
  m_b : Inport  Port=2
  mi : Inport  Port=3
  y2 : Inport  Port=4
  y4 : Inport  Port=5
  z_m : Inport  Port=6
  Constant : Constant  Value=4  OutDataTypeStr=double  SampleTime=-1
  Multiply : Product
  Multiply1 : Product
  Multiply2 : Product  Inputs=3
  Square : Math  Operator=square  SaturateOnIntegerOverflow=on
  Square1 : Math  Operator=square  SaturateOnIntegerOverflow=on
  Sum : Sum  OutDataTypeStr=double
  Sum1 : Sum
  Sum2 : Sum
  I_11 : Outport
  wires:
  Sum/1 -> I_11/1
  I_b_xx/1 -> Sum/1
  Multiply/1 -> Sum/2
  Sum1/1 -> Multiply/2
  m_b/1 -> Multiply/1
  Multiply2/1 -> Square1/1
  Square1/1 -> Sum1/2
  Square/1 -> Sum1/1
  Constant/1 -> Multiply2/3
  z_m/1 -> Multiply2/2
  y2/1 -> Sum2/1
  y4/1 -> Sum2/2
  Sum2/1 -> Multiply1/2
  Multiply1/1 -> Square/1
  mi/1 -> Multiply1/1, Multiply2/1

== system MORUS_NELINEARNI_GA_NONTILTING/MORUS/I_b_c/I_12 // I_21 ==
  m_b : Inport
  mi : Inport  Port=2
  x_1 : Inport  Port=3
  x_3 : Inport  Port=4
  y_2 : Inport  Port=5
  y_4 : Inport  Port=6
  Gain : Gain  Gain=-1
  Multiply : Product  Inputs=4
  Square : Math  Operator=square  SaturateOnIntegerOverflow=on
  Sum : Sum
  Sum1 : Sum
  I_12 : Outport
  wires:
  y_2/1 -> Sum1/1
  y_4/1 -> Sum1/2
  x_3/1 -> Sum/2
  x_1/1 -> Sum/1
  mi/1 -> Square/1
  m_b/1 -> Gain/1
  Multiply/1 -> I_12/1
  Gain/1 -> Multiply/1
  Square/1 -> Multiply/2
  Sum/1 -> Multiply/3
  Sum1/1 -> Multiply/4

== system MORUS_NELINEARNI_GA_NONTILTING/MORUS/I_b_c/I_13 // I_31 ==
  m_b : Inport
  mi : Inport  Port=2
  x_1 : Inport  Port=3
  x_3 : Inport  Port=4
  z_m : Inport  Port=5
  Constant : Constant  Value=4  OutDataTypeStr=double  SampleTime=-1
  Gain : Gain  Gain=-1
  Multiply : Product  Inputs=5
  Square : Math  Operator=square  SaturateOnIntegerOverflow=on
  Sum : Sum
  I_13 : Outport
  wires:
  z_m/1 -> Multiply/4
  x_3/1 -> Sum/2
  x_1/1 -> Sum/1
  mi/1 -> Square/1
  m_b/1 -> Gain/1
  Multiply/1 -> I_13/1
  Gain/1 -> Multiply/1
  Square/1 -> Multiply/2
  Sum/1 -> Multiply/3
  Constant/1 -> Multiply/5

== system MORUS_NELINEARNI_GA_NONTILTING/MORUS/I_b_c/I_22 ==
  I_b_yy : Inport
  m_b : Inport  Port=2
  mi : Inport  Port=3
  x_1 : Inport  Port=4
  x_3 : Inport  Port=5
  z_m : Inport  Port=6
  Constant : Constant  Value=4  OutDataTypeStr=double  SampleTime=-1
  Multiply : Product
  Multiply1 : Product
  Multiply2 : Product  Inputs=3
  Square : Math  Operator=square  SaturateOnIntegerOverflow=on
  Square1 : Math  Operator=square  SaturateOnIntegerOverflow=on
  Sum : Sum
  Sum1 : Sum
  Sum2 : Sum
  I_22 : Outport
  wires:
  Sum/1 -> I_22/1
  I_b_yy/1 -> Sum/1
  Multiply/1 -> Sum/2
  Sum1/1 -> Multiply/2
  m_b/1 -> Multiply/1
  Multiply2/1 -> Square1/1
  Square1/1 -> Sum1/2
  Square/1 -> Sum1/1
  Constant/1 -> Multiply2/3
  z_m/1 -> Multiply2/2
  x_1/1 -> Sum2/1
  x_3/1 -> Sum2/2
  Sum2/1 -> Multiply1/2
  Multiply1/1 -> Square/1
  mi/1 -> Multiply1/1, Multiply2/1

== system MORUS_NELINEARNI_GA_NONTILTING/MORUS/I_b_c/I_23 // I_32 ==
  m_b : Inport
  mi : Inport  Port=2
  y_2 : Inport  Port=3
  y_4 : Inport  Port=4
  z_m : Inport  Port=5
  Constant : Constant  Value=4  OutDataTypeStr=double  SampleTime=-1
  Gain : Gain  Gain=-1
  Multiply : Product  Inputs=5
  Square : Math  Operator=square  SaturateOnIntegerOverflow=on
  Sum : Sum
  I_23 : Outport
  wires:
  z_m/1 -> Multiply/4
  y_4/1 -> Sum/2
  y_2/1 -> Sum/1
  mi/1 -> Square/1
  m_b/1 -> Gain/1
  Multiply/1 -> I_23/1
  Gain/1 -> Multiply/1
  Square/1 -> Multiply/2
  Sum/1 -> Multiply/3
  Constant/1 -> Multiply/5

== system MORUS_NELINEARNI_GA_NONTILTING/MORUS/I_b_c/I_33 ==
  I_b_zz : Inport
  m_b : Inport  Port=2
  mi : Inport  Port=3
  y2 : Inport  Port=4
  y4 : Inport  Port=5
  x1 : Inport  Port=6
  x3 : Inport  Port=7
  Multiply : Product
  Multiply1 : Product
  Multiply2 : Product
  Square : Math  Operator=square  SaturateOnIntegerOverflow=on
  Square1 : Math  Operator=square  SaturateOnIntegerOverflow=on
  Sum{,1..3} (4 alike) : Sum
  I_33 : Outport
  wires:
  Sum/1 -> I_33/1
  I_b_zz/1 -> Sum/1
  Multiply/1 -> Sum/2
  Sum1/1 -> Multiply/2
  m_b/1 -> Multiply/1
  Multiply2/1 -> Square1/1
  Square1/1 -> Sum1/2
  Square/1 -> Sum1/1
  y2/1 -> Sum2/1
  y4/1 -> Sum2/2
  Sum2/1 -> Multiply1/2
  Multiply1/1 -> Square/1
  x3/1 -> Sum3/2
  x1/1 -> Sum3/1
  Sum3/1 -> Multiply2/2
  mi/1 -> Multiply2/1, Multiply1/1

== matlab function MORUS_NELINEARNI_GA_NONTILTING/MORUS/DOT_V_X/MATLAB Function ==
  data: u input; y output
function y = fcn(u)
if(isnan(u))
    y =0.0;
    return;
end

y = u;

== matlab function MORUS_NELINEARNI_GA_NONTILTING/MORUS/DOT_V_Y/MATLAB Function ==
  data: u input; y output
function y = fcn(u)
if(isnan(u))
    y =0.0;
    return;
end

y = u;

== matlab function MORUS_NELINEARNI_GA_NONTILTING/MPC ROLL/MATLAB Function1 ==
  settings: updateMethod=DISCRETE
  data: x0_ input size=10; u output size=4; x_ss_ input size=10; u_ss_ input size=4; kreni input size=1; A input size=10,10; B input size=10,4; R input size=4,4; R_delta input size=4,4; Q input size=10,10; samplingTime input size=1
function u  = adam(x0_, x_ss_, u_ss_, kreni, A, B, R, R_delta, Q, samplingTime)

persistent new_desire_state  pred_horizon control_horizon max_iter     ...
           scale_MV_inv  scale_OV_inv gradients gradient_past ...
           gradient_square_past gradient_past_tilda gradient_square_past_tilda ...
           x_states deriv_wrt_u epsilon rho1 rho2 delta num_heuristic_vars ...
           u_past u_current lambdas_x lambdas_u lambdas_u_ref u_horizon ref_old t u_last_step ...
           du_max u_max dead_time pred_blocking




       
if(isempty(new_desire_state) )
    u_last_step = zeros(4, 1);
    du_max = zeros(4,2);
    u_max = zeros(4,2);
    
    du_max(1,1) = samplingTime * 2;
    du_max(1,2) = -samplingTime * 2;
    du_max(2,1) = samplingTime * 2;
    du_max(2,2) = -samplingTime * 2;
    du_max(3,1) = 1*(samplingTime/0.01);
    du_max(3,2) = -1*(samplingTime/0.01);
    du_max(4,1) = 1*(samplingTime/0.01);
    du_max(4,2) = -1*(samplingTime/0.01);
    
    u_max(1,1) = 0.6 / 2 - 0.01;
    u_max(1,2) = -u_max(1,1);
    u_max(2,1) = 0.6 / 2 - 0.01;
    u_max(2,2) = -u_max(1,1);
    u_max(3,1) = 200;
    u_max(3,2) = -200;
    u_max(4,1) = 200;
    u_max(4,2) = -200;
    
    ref_old  = x_ss_;
    t = 0.0;
    epsilon = [0.03, 0.03];
	rho1 = 0.9;
	rho2 = 0.999;
	delta = 1e-7;
max_iter = 8;
% control_horizon = 30;
% pred_horizon = 50;

dead_time = 0;%5;%10
blocking =[3 4 6 6 6 10];
pred_horizon = sum(blocking);
control_horizon = length(blocking);
blocking2 = [];
for i = 1:length(blocking)
    for j = 1:blocking(i)
        blocking2 = [blocking2, i];
    end
end

pred_blocking = blocking2;
num_heuristic_vars = 2;
gradients = zeros(num_heuristic_vars*control_horizon,1 );
gradient_past = zeros(num_heuristic_vars*control_horizon,1 );
gradient_past_tilda = zeros(num_heuristic_vars*control_horizon,1 );
gradient_square_past_tilda = zeros(num_heuristic_vars*control_horizon,1 );
gradient_square_past = zeros(num_heuristic_vars*control_horizon,1 );
new_desire_state = true;
scale_OV_inv = inv(diag([0.58, 4.0, 0.58, 4.0, 800, 800, 0.5236, 0.671578600000000, 100, 100]));

scale_MV_inv = inv(diag([0.58, 0.58, 100, 100]));

% R =diag([0.67670, 0.67670, 0.13534000, 0.13534000]);
% R_delta = diag([0.738879858135067, 0.738879858135067, 0.007388798581351,0.007388798581351]);
% Q = diag([ 0.135340000000000,0.002706800000000,  0.1353400, 0.002706800, 0.002706800, 0.002706800,10.7068000, 9.676700]);

% A =[    0.4271,    0.0223,         0,         0,         0,         0,         0 ,        0;
%    -8.7243,   -0.1501,         0,         0,         0,         0,         0,         0;
%          0,         0,    0.4271,    0.0223,         0,         0,         0,         0;
%          0,         0,   -8.7243,   -0.1501,         0,         0,         0,         0;
%          0,         0,         0,         0,    0.7300,         0,         0,         0;
%          0,         0,         0,         0,         0,    0.7300,         0,         0;
%     0.0090,    0.0005,    0.0090,    0.0005,    0.0001,   -0.0001,    1.0000,    0.0787;
%     0.1699,    0.0113,    0.1699,    0.0113,    0.0028,   -0.0028,         0 ,   1.0000];
%     
% B =[ 0.5729,         0 ,        0 ,        0;
%     8.7243,         0   ,      0 ,        0;
%          0,    0.5729  ,       0 ,        0;
%          0,    8.7243 ,        0 ,        0;
%          0,         0 ,   0.2700 ,        0;
%          0,         0 ,        0 ,   0.2700;
%    -0.0037,   -0.0037,    0.0000 ,  -0.0000;
%    -0.0347,   -0.0347,    0.0005 ,  -0.0005];



x_states = zeros(size(A, 1), pred_horizon+1);
deriv_wrt_u =  zeros(size(B,2), control_horizon);
u_past = zeros(size(B,2), 1);
u_current = zeros(size(B,2), 1);
u_ss_ = zeros(size(B,2), 1);
lambdas_x = zeros(size(A, 1), pred_horizon);
lambdas_u = zeros(size(B,2), pred_horizon);
u_horizon = zeros(size(B,2), pred_horizon);
lambdas_u_ref = zeros(size(B,2), pred_horizon);

end

residuum_signal =0.0;
residuum_state =0.0;

u = zeros(size(B,2), 1);
if(kreni ~= 1)
    return;
end
x = zeros(control_horizon *num_heuristic_vars,1);
change_x = zeros(control_horizon *num_heuristic_vars,1);

if(sum(abs(x_ss_ - ref_old), 'double') < 1e-6)
   new_desire_state = false; 
else
    new_desire_state = true;
    ref_old = x_ss_;
end
new_desire_state = false; 
for iter = 1:max_iter
x_states(:,1) = x0_ ;
deriv_wrt_u = 0*deriv_wrt_u;
u_past = zeros(size(B,2), 1);% u_current*1;

if (new_desire_state) 
		new_desire_state = false;
		gradient_past = 0*gradient_past;
		gradient_square_past = 0*gradient_square_past;
		t = 0.0;
end

for i = 1:pred_horizon
    if(pred_blocking(i) <= control_horizon)
        u(1,1) = x(0*control_horizon  + pred_blocking(i));
        u(2,1) = x(0*control_horizon  + pred_blocking(i));
        u(3,1) = x(1*control_horizon  + pred_blocking(i));
        u(4,1) = -x(1*control_horizon  + pred_blocking(i));
    end
    x_states(:,i+1) = A * x_states(:,i) + B * u; 
    lambdas_x(:,i) = -1*x_ss_ + x_states(:,i+1); 
    lambdas_u(:,i) = u - u_past; 
    lambdas_u_ref(:, i) = u - u_ss_; 
    if(i>=dead_time)
        %derivation of u
        if(pred_blocking(i) <= control_horizon)
            deriv_wrt_u(:, pred_blocking(i)) = (2*R*u) -2*R*u_ss_  + (4*R_delta*u) -2*R_delta*u_past + deriv_wrt_u(:, pred_blocking(i)) ;
            
            if(i > 1)
                deriv_wrt_u(:, pred_blocking(i-1)) = deriv_wrt_u(:, pred_blocking(i-1)) -2*R_delta*u ;
            end
        else
            deriv_wrt_u(:, control_horizon) = deriv_wrt_u(:, control_horizon) + (2*R*u) -2*R*u_ss_  + (4*R_delta*u)+ (-2*R_delta*u_past) ;
            deriv_wrt_u(:, control_horizon) = deriv_wrt_u(:, control_horizon) -2*R_delta*u ;
        end
        
        %derivation of x
        for j = 1:i
            if(pred_blocking(j) <= control_horizon && pred_blocking(i) <= control_horizon)
                
                deriv_wrt_u(:,pred_blocking(j)) = deriv_wrt_u(:,pred_blocking(j)) + transpose(transpose( 2*Q*x_states(:,i+1) - 2*Q*x_ss_ )*(A^(i-j))*B);
            else
                if(j > control_horizon)
                    deriv_wrt_u(:,control_horizon) =deriv_wrt_u(:,control_horizon) +  transpose(transpose((2*Q*x_states(:,i+1) - 2*Q*x_ss_))*(A^(i-j))*B);
                else
                    deriv_wrt_u(:,pred_blocking(j)) =deriv_wrt_u(:,pred_blocking(j)) + transpose(transpose( 2*Q*x_states(:,i+1) - 2*Q*x_ss_ )*(A^(i-j))*B);
                end
            end
        end
    end
    u_past = u;
end


lambdas_u_ref =scale_MV_inv * lambdas_u_ref;
lambdas_u = scale_MV_inv * lambdas_u;
lambdas_x = scale_OV_inv * lambdas_x;
residuum_signal=sum((lambdas_u_ref.*(R*lambdas_u_ref)),'double')  + sum((lambdas_u.*(R_delta*lambdas_u)),'double'); 
residuum_state=sum((lambdas_x.*(Q*lambdas_x)),'double') ; 
        
residuum =  residuum_signal +  residuum_state;

for iter_der = 1:control_horizon
    gradients(iter_der, 1) = 2 * deriv_wrt_u(1, iter_der);
    gradients(iter_der + control_horizon, 1) = 2 * deriv_wrt_u(3, iter_der);
end

gradient_square_past = (rho2*gradient_square_past + (1 - rho2)*gradients.*(gradients));

gradient_past = (rho1*gradient_past + (1 - rho1)*gradients);

t  = t +1.0;

for adam_iter = 1:control_horizon *num_heuristic_vars
    gradient_past_tilda(adam_iter, 1) = (gradient_past(adam_iter, 1)) / (1.0 - (rho1^t));
	gradient_square_past_tilda(adam_iter, 1) = (gradient_square_past(adam_iter, 1)) / (1.0 - (rho2^t));
		

end

for h_iter = 1:num_heuristic_vars
    for c_iter = 1:control_horizon
    change_x((h_iter -1)*c_iter + c_iter, 1) = -1 * (epsilon(h_iter) * gradient_past_tilda((h_iter -1)*c_iter + c_iter, 1)) / (sqrt(gradient_square_past_tilda((h_iter -1)*c_iter + c_iter, 1)) + delta);
    end
end

x = (x + change_x);
end

u(1,1) = x(0*control_horizon  + 1);
u(2,1) = x(0*control_horizon  + 1);
u(3,1) = x(1*control_horizon  + 1);
u(4,1) = -x(1*control_horizon  + 1);

for iter_m = 1:4
    if(u(iter_m,1) > ( u_last_step(iter_m,1)+du_max(iter_m,1) ))
        u(iter_m,1) =  u_last_step(iter_m,1)+du_max(iter_m,1);
        
    elseif (u(iter_m,1) < ( u_last_step(iter_m,1)+du_max(iter_m,2) ))
        u(iter_m,1) =  u_last_step(iter_m,1)+du_max(iter_m,2);
    end
    
    if(u(iter_m,1) > u_max(iter_m,1) )
        u(iter_m,1) =  u_max(iter_m,1);
    elseif (u(iter_m,1) < u_max(iter_m,2))
        u(iter_m,1) =  u_max(iter_m,2);
    end
    
    
end
u_last_step = u;
end
